simulink model "allpass2"  (Simulink 6.6)
settings: Solver=ode45  StartTime=0.0  StopTime=10.0  RelTol=1e-3
libraries: dspsrcs4 x1, simulink_extras x1
settings Model: Creator=student  LastModifiedBy=student

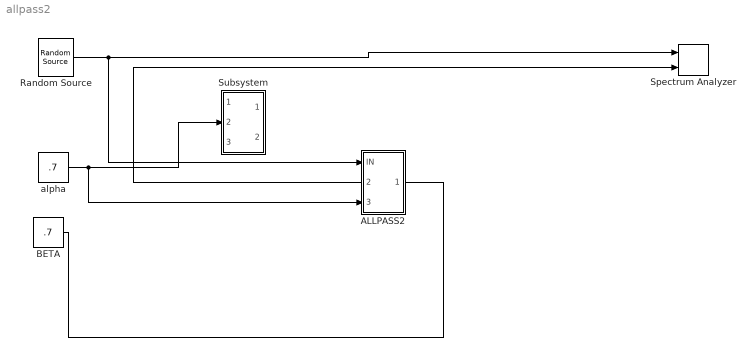
== system allpass2 ==
  ALLPASS2 : Subsystem
  BETA : Constant  Value=.7
  Random Source : dspsrcs4/Random Source  SrcType=Gaussian  NormMethod=Ziggurat  CltLength=12  MinVal=-1  MaxVal=1  MeanVal=0  VarVal=1  RepMode=Not repeatable  rawSeed=1  IsInherit=off  SampMode=Discrete  SampTime=1  SampFrame=1  DataType=Double  OutComplex=Real
  Spectrum Analyzer : simulink_extras/Additional Sinks/Spectrum Analyzer  SystemSampleTime=-1  npts=256  fftpts=256  HowOften=64  sampleT=1
  Subsystem : Subsystem
  alpha : Constant  Value=.7
  wires:
  Random Source/1 -> Spectrum Analyzer/1, ALLPASS2/1(IN)
  alpha/1 -> Subsystem/2(In2), ALLPASS2/3(ALPHA2)
  BETA/1 -> ALLPASS2/2(BETA)
  ALLPASS2/1(OUT) -> Spectrum Analyzer/2

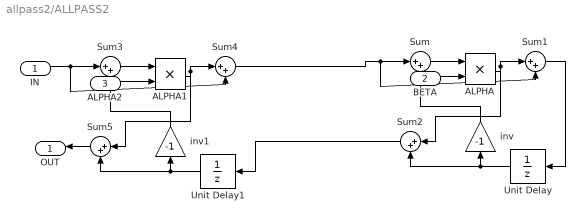
== system allpass2/ALLPASS2 ==
  IN : Inport
  BETA : Inport  Port=2
  ALPHA2 : Inport  Port=3
  ALPHA : Product  RndMeth=Zero
  ALPHA1 : Product  RndMeth=Zero
  Sum{,1,3..4} (4 alike) : Sum  Inputs=|++
  Sum2 : Sum  Orientation=left  Inputs=|++
  Sum5 : Sum  Orientation=left  Inputs=|++
  Unit Delay : UnitDelay  Orientation=left
  Unit Delay1 : UnitDelay  Orientation=left
  inv : Gain  Orientation=up  Gain=-1
  inv1 : Gain  Orientation=up  Gain=-1
  OUT : Outport  Orientation=left
  wires:
  Sum/1 -> ALPHA/1
  ALPHA/1 -> Sum1/1, Sum2/1
  Unit Delay/1 -> inv/1, Sum2/2
  inv/1 -> Sum/2
  Sum1/1 -> Unit Delay/1
  Sum2/1 -> Unit Delay1/1
  Sum3/1 -> ALPHA1/1
  ALPHA1/1 -> Sum4/1, Sum5/1
  Unit Delay1/1 -> inv1/1, Sum5/2
  inv1/1 -> Sum3/2
  Sum4/1 -> Sum/1, Sum1/2
  IN/1 -> Sum3/1, Sum4/2
  ALPHA2/1 -> ALPHA1/2
  BETA/1 -> ALPHA/2
  Sum5/1 -> OUT/1

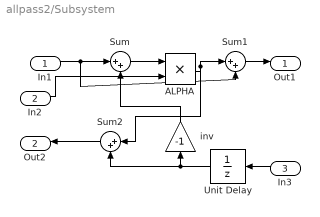
== system allpass2/Subsystem ==
  In1 : Inport
  In2 : Inport  Port=2
  In3 : Inport  Orientation=left  Port=3
  ALPHA : Product  RndMeth=Zero
  Sum : Sum  Inputs=|++
  Sum1 : Sum  Inputs=|++
  Sum2 : Sum  Orientation=left  Inputs=|++
  Unit Delay : UnitDelay  Orientation=left
  inv : Gain  Orientation=up  Gain=-1
  Out1 : Outport
  Out2 : Outport  Orientation=left  Port=2
  wires:
  Sum/1 -> ALPHA/1
  ALPHA/1 -> Sum1/1, Sum2/1
  Unit Delay/1 -> inv/1, Sum2/2
  inv/1 -> Sum/2
  In1/1 -> Sum/1, Sum1/2
  Sum1/1 -> Out1/1
  In2/1 -> ALPHA/2
  Sum2/1 -> Out2/1
  In3/1 -> Unit Delay/1
